simulink model "grade_6"  (R2025b)
settings: Solver=FixedStepAuto  StartTime=0.0  StopTime=60  FixedStep=0.01  RelTol=1e-3
model workspace (MAT data in the model file):
  freq = 0.87
settings Model: Creator=marko  LastModifiedBy=marko
settings DebuggingCC: UnconnectedInputMsg=warning  UnconnectedOutputMsg=warning  UnconnectedLineMsg=warning
settings ModelReferenceCC: EnableRefExpFcnMdlSchedulingChecks=on
settings RTWCC: GPUComputeCapability=3.5  DLArmComputeVersion=19.05

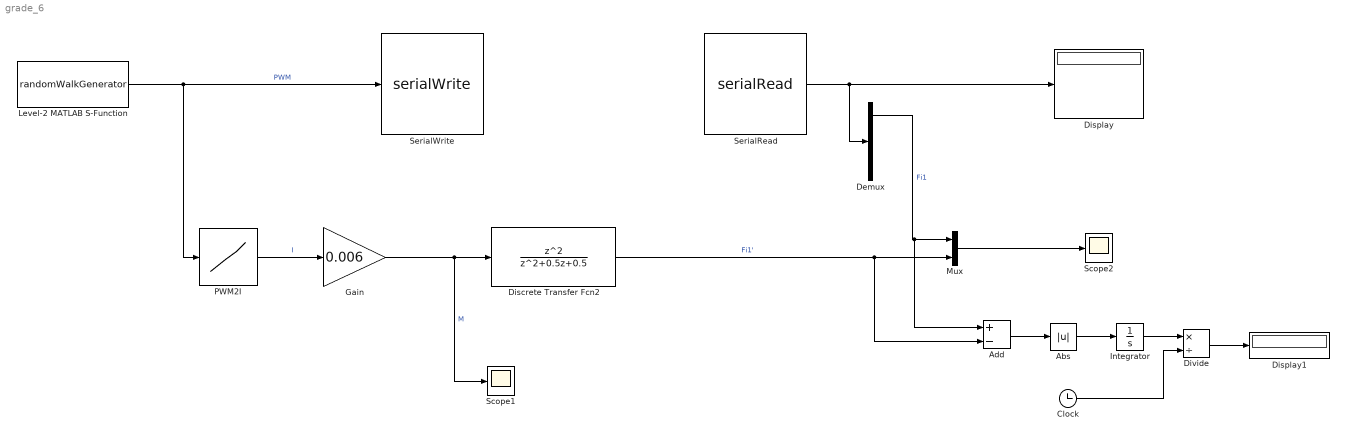
== system grade_6 ==
  Abs : Abs  SaturateOnIntegerOverflow=off
  Add : Sum  Inputs=+-
  Clock : Clock
  Demux : Demux
  Discrete Transfer Fcn2 : DiscreteTransferFcn  Numerator=[1 0 0]  Denominator=[1 0.5 0.5]
  Display : Display
  Display1 : Display
  Divide : Product  Inputs=*/
  Gain : Gain  Gain=0.006
  Integrator : Integrator
  Level-2 MATLAB S-Function : M-S-Function  FunctionName=randomWalkGenerator
  Mux : Mux  Inputs=2
  PWM2I : Lookup_n-D  NumberOfTableDimensions=1  BreakpointsForDimension1=|  Table=|  InternalRulePriority=Speed  RndMeth=Simplest
      BreakpointsForDimension1=|
      | [ ...
      |    -4000; -3875; -3750; -3625; -3500; -3375; -3250; -3125; ...
      |    -3000; -2875; -2750; -2625; -2500; -2375; -2250; -2125; ...
      |    -2000; -1875; -1750; -1625; -1500; -1375; -1250; -1125; ...
      |    -1000;  -875;  -750;  -625;  -500;  -375;  -250;  -125; ...
      |        0; ...
      |      125;   250;   375;   500;   625;   750;   875;  1000; ...
      |     1125;  1250;  1375;  1500;  1625;  1750;  1875;  2000; ...
      |     2125;  2250;  2375;  2500;  2625;  2750;  2875;  3000; ...
      |     3125;  3250;  3375;  3500;  3625;  3750;  3875;  4000  ...
      | ]
      Table=|
      | [ ...
      |    -1.0346; -1.0331; -1.0334; -1.0337; -1.0310; -1.0314; -1.0297; -1.0293; ...
      |    -1.0298; -1.0276; -1.0263; -1.0253; -1.0241; -1.0237; -1.0225; -1.0194; ...
      |    -1.0188; -1.0142; -1.0117; -1.0059; -1.0031; -0.9984; -0.9934; -0.9842; ...
      |    -0.9693; -0.9515; -0.9373; -0.9088; -0.8800; -0.8097; -0.6768;  0.0000; ...
      |     0.0000; ...
      |     0.0000;  0.0000;  0.5970;  0.7090;  0.7996;  0.8580;  0.9030;  0.9253; ...
      |     0.9417;  0.9608;  0.9725;  0.9807;  0.9874;  0.9956;  1.0006;  1.0035; ...
      |     1.0095;  1.0121;  1.0126;  1.0158;  1.0181;  1.0181;  1.0185;  1.0202; ...
      |     1.0217;  1.0219;  1.0243;  1.0251;  1.0249;  1.0144;  1.0082;  1.0080  ...
      | ]
  Scope1 : Scope
      settings: ActiveDisplayYMinimum=-0.0060867  ActiveDisplayYMaximum=0.0030599
  Scope2 : Scope
      settings: ActiveDisplayYMinimum=-0.0060867  ActiveDisplayYMaximum=0.0030599  DataLoggingVariableName=ScopeData2
  SerialRead : M-S-Function  FunctionName=serialRead  Parameters='COM4'
  SerialWrite : M-S-Function  FunctionName=serialWrite  Parameters='COM4'
  wires:
  SerialRead/1 -> Demux/1, Display/1
  Level-2 MATLAB S-Function/1 -> PWM2I/1, SerialWrite/1  "PWM"
  Demux/1 -> Add/1, Mux/1  "Fi1"
  Mux/1 -> Scope2/1
  Gain/1 -> Scope1/1, Discrete Transfer Fcn2/1  "M"
  PWM2I/1 -> Gain/1  "I"
  Discrete Transfer Fcn2/1 -> Add/2, Mux/2  "Fi1'"
  Add/1 -> Abs/1
  Abs/1 -> Integrator/1
  Integrator/1 -> Divide/1
  Divide/1 -> Display1/1
  Clock/1 -> Divide/2
